simulink model "main_sim_adapt_Gref_SP"  (Simulink 7.2)
settings: Solver=ode2  SolverMode=SingleTasking  StartTime=0.0  StopTime=tsim_max  FixedStep=dtsim  RelTol=1e-3
StopFcn:
  | %mkplt
values from neighbouring files (symbols this model uses):
  aero_surf_qbar_off = get_value('aero_surf_qbar_off')    [setup_claw.m]
  aero_surf_qbar_on = get_value('aero_surf_qbar_on')    [setup_claw.m]
  assertion_time = get_value('assertion_time')    [setup_sim.m]
  att_cmd_select = get_value('att_cmd_select')    [setup_sim.m]
  att_trim_IC = orientation.att'    [setup_claw.m]
  att_type_numbers = cell2mat(struct2cell(att_type))    [setup_constants.m]
  chi_trim_IC = orientation.Vchigam(2)    [setup_claw.m]
  command_time = engage_time + 2.0    [setup_sim.m]
  compute_all_rate_cols = get_value('compute_all_rate_cols')    [setup_claw.m]
  compute_all_vel_cols = get_value('compute_all_vel_cols')    [setup_claw.m]
  da_trim_IC = tmp(1)    [setup_claw.m]
  dc_L2W_IC = orientation.dc_L2W    [setup_claw.m]
  de_trim_IC = tmp(2)    [setup_claw.m]
  dr_trim_IC = tmp(3)    [setup_claw.m]
  dtsim = get_value('dtsim')    [setup_sim.m]
  E_trim_IC = MACH_pos_IC(2)    [setup_claw.m]
  Ed_trim_IC = MACH_vel_IC(2)    [setup_claw.m]
  gain_set = gain_set_next    (= 1)    [setup_claw.m]
  gain_var_struct = rmfield(gain_var_struct,setdiff(fieldnames(gain_var_struct),{'name','size'}))    [setup_claw.m]
  gamma_trim_IC = orientation.Vchigam(3)    [setup_claw.m]
  h_trim_IC = MACH_pos_IC(3)    [setup_claw.m]
  hd_trim_IC = MACH_vel_IC(3)    [setup_claw.m]
  ideal_vel_Kb = MACH_vel_Kb(1)    [setup_sim.m]
  MACH = rmfield(MACH,'vel_throt_lrlim')    [setup_claw.m]
  MACH_att_fb = get_value('MACH_att_fb','onerror',0)    [setup_claw.m]
  MACH_att_int_IC = (1-MACH_att_Kc).*MACH_quat_IC'    [setup_ideal.m]
  MACH_att_Kb = repval(att_kbnom,MACH.att_num_cv)    [setup_claw.m]
  MACH_att_Kc = Ki2Kc(MACH_att_Ki)    [setup_ideal.m]
  MACH_att_Ki = repval(att_fi,MACH.att_num_cv)    [setup_claw.m]
  MACH_gain_mat = vertcat(MACH_gain_mat, this_gain_mat)    [setup_claw.m]
  MACH_mass_IC = obac_params.mass_IC    [setup_claw.m]
  MACH_pos_IC = x_obac_IC(MACH.NEh_idx)    [setup_claw.m]
  MACH_pos_int_IC = (1-MACH_pos_Kc).*MACH_pos_IC' + MACH_vel_IC'./MACH_pos_Kb    [setup_ideal.m]
  MACH_pos_Kb = repval(pos_kbnom,MACH.pos_num_cv)    [setup_claw.m]
  MACH_pos_Kc = Ki2Kc(MACH_pos_Ki)    [setup_ideal.m]
  MACH_pos_Ki = repval(pos_fi,MACH.pos_num_cv)    [setup_claw.m]
  MACH_pqr_Bmat_IC = Bo(MACH.pqr_idx,MACH.pqr_u_idx)    [setup_claw.m]
  MACH_pqr_IC = pqr_trim_IC    [setup_claw.m]
  MACH_pqr_int_IC = (1-MACH_pqr_Kc).*MACH_pqr_IC'    [setup_ideal.m]
  MACH_pqr_Kb = repval(pqr_kbnom,MACH.pqr_num_cv)    [setup_claw.m]
  MACH_pqr_Kc = Ki2Kc(MACH_pqr_Ki)    [setup_ideal.m]
  MACH_pqr_Ki = repval(pqr_fi,MACH.pqr_num_cv)    [setup_claw.m]
  MACH_pqr_u_IC = [ vanes_trim_IC; tvc_trim_IC; rcs_trim_IC ]    [setup_claw.m]
  MACH_quat_IC = quat_trim_IC    [setup_claw.m]
  MACH_throttle_IC = throttle_trim_IC    [setup_claw.m]
  MACH_U_nom_IC = zeros(MACH.num_u,1)    [setup_claw.m]
  MACH_vel_Bmat_IC = MACH_vel_Bmat_IC*inv(vel_perts)    [setup_claw.m]
  MACH_vel_cvdnom_IC = repval(get_value('vel_cvdnom_IC','onerror',MACH_vel_cvdnom_IC),length(MACH_vel_cvdnom_IC))'    [setup_claw.m]
  MACH_vel_IC = orientation.NdEdhd'    [setup_claw.m]
  MACH_vel_int_IC = (1-MACH_vel_Kc).*MACH_vel_IC'    [setup_ideal.m]
  MACH_vel_Kb = repval(vel_kbnom,MACH.vel_num_cv)    [setup_claw.m]
  MACH_vel_Kc = Ki2Kc(MACH_vel_Ki)    [setup_ideal.m]
  MACH_vel_Ki = repval(vel_fi,MACH.vel_num_cv)    [setup_claw.m]
  MACH_vel_uold_IC = [ MACH_quat_IC; MACH_throttle_IC ]    [setup_claw.m]
  N_trim_IC = MACH_pos_IC(1)    [setup_claw.m]
  Nd_trim_IC = MACH_vel_IC(1)    [setup_claw.m]
  obac_params = define_model('obac', get_value('obac_model_type'))    [setup_claw.m]
  pos_cmd_select = get_value('pos_cmd_select')    [setup_sim.m]
  pqr_trim_IC = [ 0 0 0 ]'    [setup_claw.m]
  rate_cmd_select = get_value('rate_cmd_select')    [setup_sim.m]
  rcs_cvddes_thresh = get_value('rcs_cvddes_thresh')    [setup_claw.m]
  reset_camcmd_on_entry = get_value('reset_camcmd_on_entry')    [setup_claw.m]
  throttle_trim_IC = u_obac_IC(MACH.throttle_idx)    [setup_claw.m]
  trac_params = define_model('trac', get_value('trac_model_type','onerror',obac_params.model_type))    [setup_sim.m]
  use_auto_att_type = get_value('use_auto_att_type','onerror',0)    [setup_claw.m]
  use_eow_as_iv = get_value('use_eow_as_iv')    [setup_claw.m]
  use_full_surf_cmd = get_value('use_full_surf_cmd')    [setup_sim.m]
  use_nav = get_value('use_nav')    [setup_claw.m]
  use_NdEdh_pos = get_value('use_NdEdh_pos')    [setup_claw.m]
  use_pos_fltpath_lim = get_value('use_pos_fltpath_lim')    [setup_claw.m]
  use_throt_estimate = get_value('use_throt_estimate')    [setup_claw.m]
  use_variable_mass = get_value('use_variable_mass')    [setup_claw.m]
  use_wind_est = get_value('use_wind_est')    [setup_claw.m]
  V_trim_IC = orientation.Vchigam(1)    [setup_claw.m]
  vel_cmd_ramp_time = get_value('vel_cmd_ramp_time')    [setup_claw.m]
  vel_cmd_select = get_value('vel_cmd_select')    [setup_sim.m]
  x_trac_IC = x_obac_IC    [setup_sim.m]
undefined symbols (not defined in the file or in its folder): accel_cmd, alpha_trim, Am, att_type, B1, bb_ellipsoid, bb_params, Bm, C, constants, cosA, DiscIntNeverNeededParam, DZkx, DZtheta, E_rwy, Ed_cmd, eow_boundary, flag_autoadapt, flag_exsig, flag_uad, full_surf_llim, full_surf_ulim, gam_cmd_descent, gam_cmd_preflare, gamdot_cmd_descent, gamdot_cmd_flare, gamdot_cmd_preflare, Gamtheta, Gamx, hd_cmd, in_error_thresh, in_exsig_vecin, in_exsig_vecout, in_reset_stoptime, in_t_exsig, in_t_timer, in_tadaptoff_forced, in_tadapton_forced, Kb, Kxhat0, Kxnom, Kxstar, max_chi_cmd, max_LOS_rate, max_vel_cmd, min_chi_cmd, min_vel_cmd, modes, N_rwy, Nd_cmd, Nrbf, P, pos, Sig, sinA, target_pos_IC, target_range_blind, target_range_detect, target_range_homing, target_vel_IC ... (+11)
libraries: simulink x44, utility_lib x36, mach_lib x24, model_lib x13, simulink_need_slupdate x8, models x8
(part 1 of 8)
CloseFcn:
  | rtwprivate ssgencode ModelCloseRequest main
settings Model: Creator=E183308  LastModifiedBy=E183308  ModifiedComment=E700252 -- Tue Nov 11 13:33:23 2003 -- Version 1.2477  TunableVars=MACH_U_nom_IC,MACH_gain_mat,MACH_mass_IC,MACH_pos_IC,MACH_pqr_Bmat_IC,MACH_pqr_u_IC,MACH_quat_IC,MACH_throttle_IC,MACH_vel_Bmat_IC,MACH_vel_IC,MACH_vel_cvdnom_IC,MACH_vel_uold_IC  TunableVarsStorageClass=Auto,Auto,Auto,Auto,Auto,Auto,Auto,Auto,Auto,Auto,Auto,Auto  TunableVarsTypeQualifier=,,,,,,,,,,,  BufferReuse=off
settings DataIOCC: LimitDataPoints=off  SaveOutput=off  SaveTime=off  SignalLoggingName=sigsOut
settings OptimizationCC: BlockReduction=off  BooleanDataType=off  BufferReuse=off  EnforceIntegerDowncast=off  FoldNonRolledExpr=off  InitFltsAndDblsToZero=on
settings DebuggingCC: SaveWithParameterizedLinksMsg=none  SignalResolutionControl=TryResolveAllWithWarning  SolverPrmCheckMsg=none  InheritedTsInSrcMsg=none  MultiTaskDSMMsg=warning  MultiTaskCondExecSysMsg=none  StrictBusMsg=ErrorLevel1
settings HardwareCC: TargetEndianess=LittleEndian  TargetHWDeviceType=MATLAB Host  ProdEqTarget=off
settings SFSimCC: SFSimEcho=off
settings RTWCC: SystemTargetFile=rtwsfcn.tlc  TemplateMakefile=rtwsfcn_default_tmf  Description=S-function Target  ProcessScript=rtwsfcn_make_rtw_hook  IncludeERTFirstTime=on
settings STFCustomTargetCC: TargetFcnLib=ansi_tfl_tmw.mat  ModelReferenceCompliant=off  SystemTargetFile=rtwsfcn.tlc
settings CustomProperty: Value=on

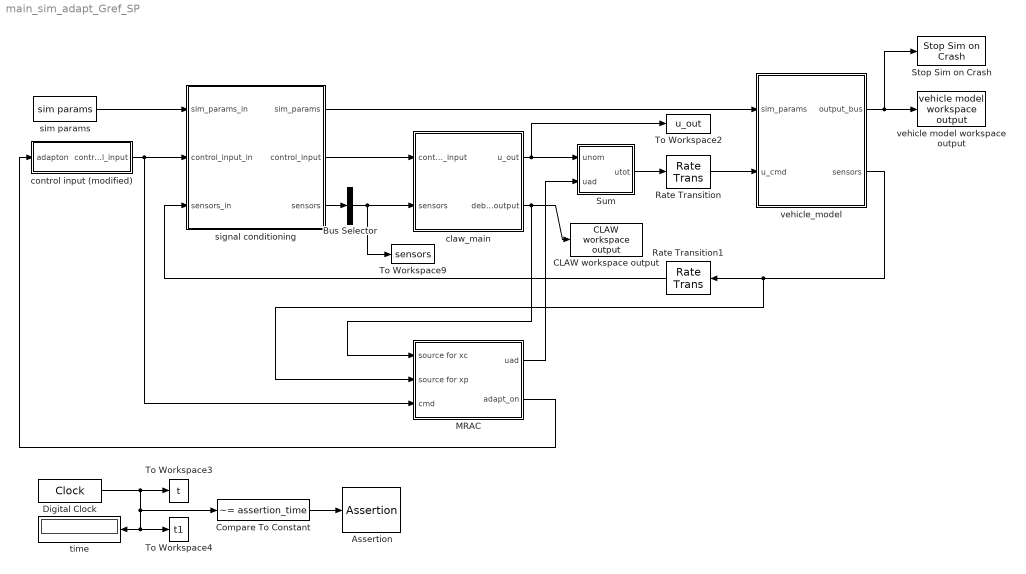
== system main_sim_adapt_Gref_SP ==
  Assertion : Assertion  Enabled=on  AssertionFailFcn=assertioncb  StopWhenAssertionFail=off
  Bus Selector : BusSelector  OutputSignals=pqr,NED_dot,latlonh,e,accels_cg,nav_ok,u_meas,NED_wind,seeker  OutputAsBus=on
  CLAW workspace output : mach_lib/CLAW workspace output  SystemSampleTime=-1
  Compare To Constant : simulink/Logic and Bit Operations/Compare To Constant  SystemSampleTime=-1  relop=~=  const=assertion_time  LogicOutDataTypeMode=boolean  ZeroCross=off
  Digital Clock : DigitalClock  SampleTime=dtsim
  MRAC : Subsystem  SystemSampleTime=dtsim
  Rate Transition : RateTransition  X0=MACH_U_nom_IC
  Rate Transition1 : RateTransition  Orientation=left  OutPortSampleTime=MACH.dt
  Stop Sim on Crash : mach_lib/Stop Sim on Crash  SystemSampleTime=-1
  Sum : Subsystem
  To Workspace2 : ToWorkspace  VariableName=u_out  SampleTime=MACH.dt  SaveFormat=Array
  To Workspace3 : ToWorkspace  VariableName=t  SampleTime=dtsim  SaveFormat=Array
  To Workspace4 : ToWorkspace  VariableName=t1  SampleTime=MACH.dt  SaveFormat=Array
  To Workspace9 : ToWorkspace  VariableName=sensors  SampleTime=MACH.dt  SaveFormat=Array
      settings: MaxDataPoints=Inf
  claw_main : Subsystem  AncestorBlock=mach_lib/claw_main  TreatAsAtomicUnit=on  SystemSampleTime=MACH.dt
  control input (modified) : Subsystem
  signal conditioning : Subsystem
  sim params : mach_lib/sim params  SystemSampleTime=-1
  time : Display
  vehicle model workspace output : mach_lib/vehicle model workspace output  SystemSampleTime=-1
  vehicle_model : Subsystem  TreatAsAtomicUnit=on
  wires:
  Digital Clock/1 -> To Workspace3/1, Compare To Constant/1, time/1, To Workspace4/1
  claw_main/1(u_out) -> Sum/1(unom), To Workspace2/1
  vehicle_model/2(sensors) -> Rate Transition1/1, MRAC/2(source for xp)
  claw_main/2(debug_output) -> CLAW workspace output/1, MRAC/1(source for xc)
  Rate Transition/1 -> vehicle_model/2(u_cmd)
  Bus Selector/1 -> To Workspace9/1, claw_main/2(sensors)
  vehicle_model/1(output_bus) -> vehicle model workspace output/1, Stop Sim on Crash/1
  Rate Transition1/1 -> signal conditioning/3(sensors_in)
  signal conditioning/3(sensors) -> Bus Selector/1
  signal conditioning/2(control_input) -> claw_main/1(control_input)
  sim params/1 -> signal conditioning/1(sim_params_in)
  signal conditioning/1(sim_params) -> vehicle_model/1(sim_params)
  Compare To Constant/1 -> Assertion/1
  MRAC/1(uad) -> Sum/2(uad)
  Sum/1(utot) -> Rate Transition/1
  control input (modified)/1(control_input) -> signal conditioning/2(control_input_in), MRAC/3(cmd)
  MRAC/2(adapt_on) -> control input (modified)/1(adapton)

== system main_sim_adapt_Gref_SP/MRAC ==
  source for xc : Inport
  source for xp : Inport  Port=2
  cmd : Inport  Port=3
  Bus Selector1 : BusSelector  OutputSignals=command  OutputAsBus=on
  Constant : Constant  Value=flag_autoadapt  OutDataType=sfix(16)  OutScaling=2^0
  Enable Adaptation : Subsystem
  Estimate of x : Subsystem
  Force Adaptation : Subsystem
  Model Reference Adaptive Control : Subsystem
  Ref Model : Subsystem
  Reshape : Reshape  OutputDimensionality=Column vector (2-D)
  Selector : Selector  InputPortWidth=4  IndexOptions=Index vector (dialog)  Indices=[2]  OutputSizes=1
  Sum : Sum  Inputs=-|+  OutDataType=sfix(16)  OutScaling=2^0
  Switch : Switch  Threshold=0.5  OutDataType=sfix(16)  OutScaling=2^0
  Terminator : Terminator
  Terminator1 : Terminator
  To Workspace1 : ToWorkspace  VariableName=uad_xm  SampleTime=MACH.dt  SaveFormat=Array
  To Workspace2 : ToWorkspace  VariableName=uad_conv  SampleTime=MACH.dt  SaveFormat=Array
  To Workspace3 : ToWorkspace  VariableName=uad_x  SampleTime=MACH.dt  SaveFormat=Array
  adapt_onoff : Scope
      settings: SaveName=ScopeData26
  command : Scope
      settings: YMin=0  YMax=15  SaveName=ScopeData6
  uad out : Scope
      settings: SaveName=ScopeData15
  uad : Outport  OutDataType=sfix(16)  OutScaling=2^0
  adapt_on : Outport  Port=2  OutDataType=sfix(16)  OutScaling=2^0
  wires:
  Bus Selector1/1 -> Selector/1, Model Reference Adaptive Control/4(r), command/1
  Selector/1 -> Ref Model/2(r)
  cmd/1 -> Bus Selector1/1
  Model Reference Adaptive Control/1(uad) -> uad out/1, uad/1
  Model Reference Adaptive Control/3(Kx_hat) -> Terminator/1
  Model Reference Adaptive Control/4(Theta_hat) -> Terminator1/1
  source for xp/1 -> Estimate of x/2(In2)
  source for xc/1 -> Estimate of x/1(In1)
  Estimate of x/1(x) -> Sum/2, Model Reference Adaptive Control/3(x), Reshape/1, Ref Model/3(x)
  Sum/1 -> Model Reference Adaptive Control/2(e), Enable Adaptation/1(e)
  Model Reference Adaptive Control/2(uad_conv) -> To Workspace2/1
  Ref Model/1(xm) -> Sum/1, To Workspace1/1
  Enable Adaptation/1(adapt on-off) -> Switch/1
  Constant/1 -> Switch/2
  Force Adaptation/1(adapt on-off (forced)) -> Switch/3
  Switch/1 -> Model Reference Adaptive Control/1(adapt on-off), adapt_on/1, adapt_onoff/1, Ref Model/1(enable)
  Reshape/1 -> To Workspace3/1

== system main_sim_adapt_Gref_SP/Sum ==
  unom : Inport
  uad : Inport  Port=2
  Rate Transition1 : RateTransition  OutPortSampleTime=MACH.dt
  Sum : Sum  Inputs=|++  OutDataType=sfix(16)  OutScaling=2^0
  To Workspace1 : ToWorkspace  VariableName=elev_nom  SampleTime=MACH.dt  SaveFormat=Array
  To Workspace2 : ToWorkspace  VariableName=elev_adap  SampleTime=MACH.dt  SaveFormat=Array
  To Workspace9 : ToWorkspace  VariableName=elev_total  SampleTime=MACH.dt  SaveFormat=Array
  get RIE : Selector  InputPortWidth=MACH.num_u  IndexOptions=Index vector (dialog)  Indices=MACH.u_idx.elev  OutputSizes=1
  set RIE : Assignment  IndexOptions=Index vector (dialog)  Indices=MACH.u_idx.elev  OutputSizes=[1 1]
  utot : Outport
  wires:
  unom/1 -> get RIE/1, set RIE/1
  get RIE/1 -> Sum/1, To Workspace1/1
  uad/1 -> Rate Transition1/1
  Sum/1 -> set RIE/2, To Workspace9/1
  set RIE/1 -> utot/1
  Rate Transition1/1 -> To Workspace2/1, Sum/2

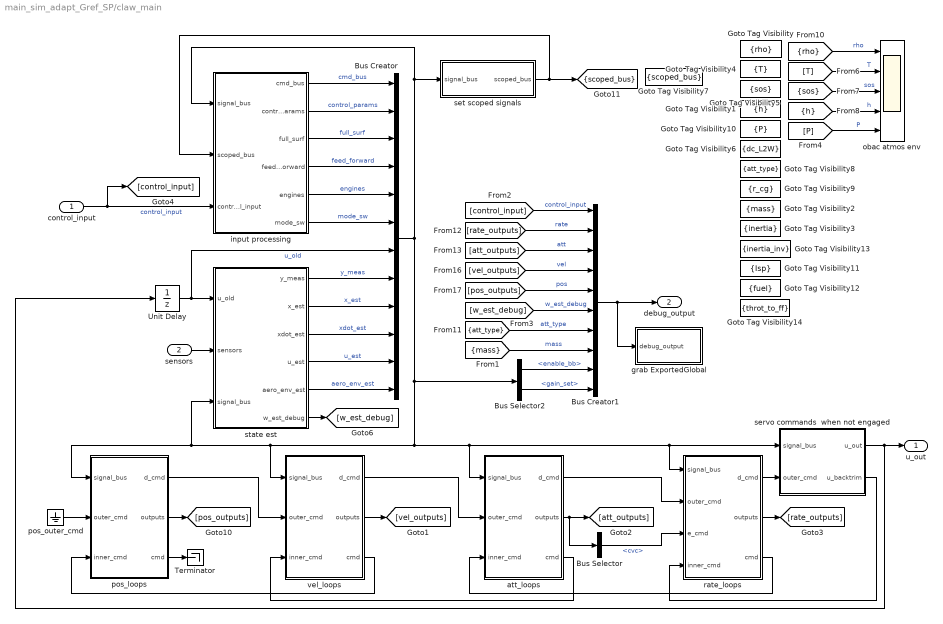
== system main_sim_adapt_Gref_SP/claw_main ==
  control_input : Inport  OutDataType=sfix(16)  OutScaling=2^0
      settings: BusObject=control_input_bus
  sensors : Inport  Port=2  OutDataType=sfix(16)  OutScaling=2^0
  Bus Creator : BusCreator  Inputs=12
  Bus Creator1 : BusCreator  Inputs=10
      settings: BusObject=CLAW_DEBUG_OUTPUT_BUS
  Bus Selector : BusSelector  OutputSignals=cvc
  Bus Selector2 : BusSelector  OutputSignals=control_params.enable_bb,control_params.gain_set
  Goto Tag Visibility : GotoTagVisibility  GotoTag=rho
  Goto Tag Visibility1 : GotoTagVisibility  GotoTag=h
  Goto Tag Visibility10 : GotoTagVisibility  GotoTag=P
  Goto Tag Visibility11 : GotoTagVisibility  GotoTag=Isp
  Goto Tag Visibility12 : GotoTagVisibility  GotoTag=fuel
  Goto Tag Visibility13 : GotoTagVisibility  GotoTag=inertia_inv
  Goto Tag Visibility14 : GotoTagVisibility  GotoTag=throt_to_ff
  Goto Tag Visibility2 : GotoTagVisibility  GotoTag=mass
  Goto Tag Visibility3 : GotoTagVisibility  GotoTag=inertia
  Goto Tag Visibility4 : GotoTagVisibility  GotoTag=T
  Goto Tag Visibility5 : GotoTagVisibility  GotoTag=sos
  Goto Tag Visibility6 : GotoTagVisibility  GotoTag=dc_L2W
  Goto Tag Visibility7 : GotoTagVisibility  GotoTag=scoped_bus
  Goto Tag Visibility8 : GotoTagVisibility  GotoTag=att_type
  Goto Tag Visibility9 : GotoTagVisibility  GotoTag=r_cg
  Terminator : Terminator
  Unit Delay : UnitDelay  X0=MACH_U_nom_IC  SampleTime=-1
  att_loops : Subsystem
  grab ExportedGlobal : Subsystem
  input processing : Subsystem
  obac atmos env : Scope  NumInputPorts=5
      settings: YMin=-5~-5~-5~-5~-5  YMax=5~5~5~5~5  SaveName=ScopeData2
  pos_loops : Subsystem
      settings: RTWSystemCode=Function
  pos_outer_cmd : Ground
  rate_loops : Subsystem
      settings: RTWSystemCode=Function
  servo commands  when not engaged : Subsystem
  set scoped signals : Subsystem
  state est : Subsystem
  vel_loops : Subsystem
      settings: RTWSystemCode=Function
  u_out : Outport  OutDataType=sfix(16)  OutScaling=2^0
  debug_output : Outport  Port=2  OutDataType=sfix(16)  OutScaling=2^0
  tag scope: scoped_bus=scoped
  wires:
  input processing/6(mode_sw) -> Bus Creator/6  "mode_sw"
  input processing/5(engines) -> Bus Creator/5  "engines"
  pos_loops/2(outputs) -> [pos_outputs]
  [pos_outputs] -> Bus Creator1/5  "pos"
  [vel_outputs] -> Bus Creator1/4  "vel"
  [att_outputs] -> Bus Creator1/3  "att"
  [rate_outputs] -> Bus Creator1/2  "rate"
  att_loops/1(d_cmd) -> rate_loops/2(outer_cmd)
  vel_loops/1(d_cmd) -> att_loops/2(outer_cmd)
  rate_loops/1(d_cmd) -> servo commands  when not engaged/2(outer_cmd)
  Bus Creator/1 -> att_loops/1(signal_bus), rate_loops/1(signal_bus), servo commands  when not engaged/1(signal_bus), vel_loops/1(signal_bus), pos_loops/1(signal_bus), state est/3(signal_bus), Bus Selector2/1, input processing/1(signal_bus), set scoped signals/1(signal_bus)
  pos_loops/3(cmd) -> Terminator/1
  att_loops/3(cmd) -> vel_loops/3(inner_cmd)
  rate_loops/3(cmd) -> att_loops/3(inner_cmd)
  pos_loops/1(d_cmd) -> vel_loops/2(outer_cmd)
  vel_loops/2(outputs) -> [vel_outputs]
  att_loops/2(outputs) -> [att_outputs], Bus Selector/1
  rate_loops/2(outputs) -> [rate_outputs]
  Bus Creator1/1 -> debug_output/1, grab ExportedGlobal/1(debug_output)
  Unit Delay/1 -> state est/1(u_old), Bus Creator/7  "u_old"
  sensors/1 -> state est/2(sensors)
  vel_loops/3(cmd) -> pos_loops/3(inner_cmd)
  servo commands  when not engaged/2(u_backtrim) -> rate_loops/4(inner_cmd)
  state est/4(u_est) -> Bus Creator/11  "u_est"
  state est/3(xdot_est) -> Bus Creator/10  "xdot_est"
  state est/2(x_est) -> Bus Creator/9  "x_est"
  state est/1(y_meas) -> Bus Creator/8  "y_meas"
  servo commands  when not engaged/1(u_out) -> u_out/1, Unit Delay/1
  pos_outer_cmd/1 -> pos_loops/2(outer_cmd)
  state est/6(w_est_debug) -> [w_est_debug]
  [w_est_debug] -> Bus Creator1/6  "w_est_debug"
  [att_type] -> Bus Creator1/7  "att_type"
  input processing/2(control_params) -> Bus Creator/2  "control_params"
  [h] -> obac atmos env/4  "h"
  [sos] -> obac atmos env/3  "sos"
  [T] -> obac atmos env/2  "T"
  [rho] -> obac atmos env/1  "rho"
  [P] -> obac atmos env/5  "P"
  state est/5(aero_env_est) -> Bus Creator/12  "aero_env_est"
  input processing/3(full_surf) -> Bus Creator/3  "full_surf"
  input processing/4(feed_forward) -> Bus Creator/4  "feed_forward"
  set scoped signals/1(scoped_bus) -> [scoped_bus], input processing/2(scoped_bus)
  [mass] -> Bus Creator1/8  "mass"
  Bus Selector2/1 -> Bus Creator1/9  "<enable_bb>"
  Bus Selector2/2 -> Bus Creator1/10  "<gain_set>"
  control_input/1 -> input processing/3(control_input), [control_input]  "control_input"
  input processing/1(cmd_bus) -> Bus Creator/1  "cmd_bus"
  [control_input] -> Bus Creator1/1  "control_input"
  Bus Selector/1 -> rate_loops/3(e_cmd)  "<cvc>"

== system main_sim_adapt_Gref_SP/control input (modified) ==
  adapton : Inport
  Add Excitation : Subsystem
  Bus Assignment : BusAssignment  AssignedSignals=command
  control input : Subsystem  AncestorBlock=mach_lib/control input  SystemSampleTime=MACH.dt
  ideal responses : Subsystem  AncestorBlock=model_lib/ideal responses
  control_input : Outport
  wires:
  Bus Assignment/1 -> ideal responses/1(control_input), control_input/1
  Add Excitation/1(Out) -> Bus Assignment/2
  control input/1(control_input) -> Add Excitation/1(In), Bus Assignment/1
  adapton/1 -> Add Excitation/2(Adapt On-Off)

== system main_sim_adapt_Gref_SP/signal conditioning ==
  sim_params_in : Inport  OutDataType=sfix(16)  OutScaling=2^0
  control_input_in : Inport  Port=2  OutDataType=sfix(16)  OutScaling=2^0
  sensors_in : Inport  Port=3  OutDataType=sfix(16)  OutScaling=2^0
  Bus Assignment : BusAssignment  AssignedSignals=full_surf.full_surf_pref
  Bus Selector : BusSelector  OutputSignals=full_surf.full_surf_pref
  Compare To Constant : simulink/Logic and Bit Operations/Compare To Constant  SystemSampleTime=-1  relop=>=  const=0  LogicOutDataTypeMode=boolean  ZeroCross=off
  Compare To Constant1 : simulink/Logic and Bit Operations/Compare To Constant  SystemSampleTime=-1  relop=<=  const=5  LogicOutDataTypeMode=boolean  ZeroCross=off
  Constant : Constant  Value=360  OutDataType=sfix(16)  OutScaling=2^0
  Digital Clock : DigitalClock  SampleTime=MACH.dt
  Gain : Gain  Gain=0  ParameterDataType=sfix(16)  ParameterScaling=2^0  OutDataType=sfix(16)  OutScaling=2^0
  Logical Operator : Logic  AllPortsSameDT=off
  Product : Product  OutDataType=sfix(16)  OutScaling=2^0  RndMeth=Zero
  Sine Wave : Sin  TimeSource=Use external signal  Amplitude=5  Frequency=2*pi  SampleTime=0
  Sum : Sum  Inputs=|++  OutDataType=sfix(16)  OutScaling=2^0
  Sum1 : Sum  Inputs=|+-  OutDataType=sfix(16)  OutScaling=2^0
  get RIE : Selector  InputPortWidth=MACH.num_u  IndexOptions=Index vector (dialog)  Indices=MACH.vane_idx(1)  OutputSizes=1
  set RIE : Assignment  IndexOptions=Index vector (dialog)  Indices=MACH.vane_idx(1)  OutputSizes=[1 1]
  sim_params : Outport  OutDataType=sfix(16)  OutScaling=2^0
  control_input : Outport  Port=2  OutDataType=sfix(16)  OutScaling=2^0
  sensors : Outport  Port=3  OutDataType=sfix(16)  OutScaling=2^0
  wires:
  sim_params_in/1 -> sim_params/1
  control_input_in/1 -> Bus Assignment/1, Bus Selector/1
  sensors_in/1 -> sensors/1
  set RIE/1 -> Bus Assignment/2
  Sum/1 -> set RIE/2
  Bus Selector/1 -> set RIE/1, get RIE/1  "<full_surf_pref>"
  get RIE/1 -> Sum/1
  Digital Clock/1 -> Sum1/1
  Constant/1 -> Sum1/2
  Sum1/1 -> Sine Wave/1, Compare To Constant/1, Compare To Constant1/1
  Compare To Constant/1 -> Logical Operator/1
  Compare To Constant1/1 -> Logical Operator/2
  Logical Operator/1 -> Product/2
  Sine Wave/1 -> Product/1
  Product/1 -> Gain/1
  Bus Assignment/1 -> control_input/1
  Gain/1 -> Sum/2

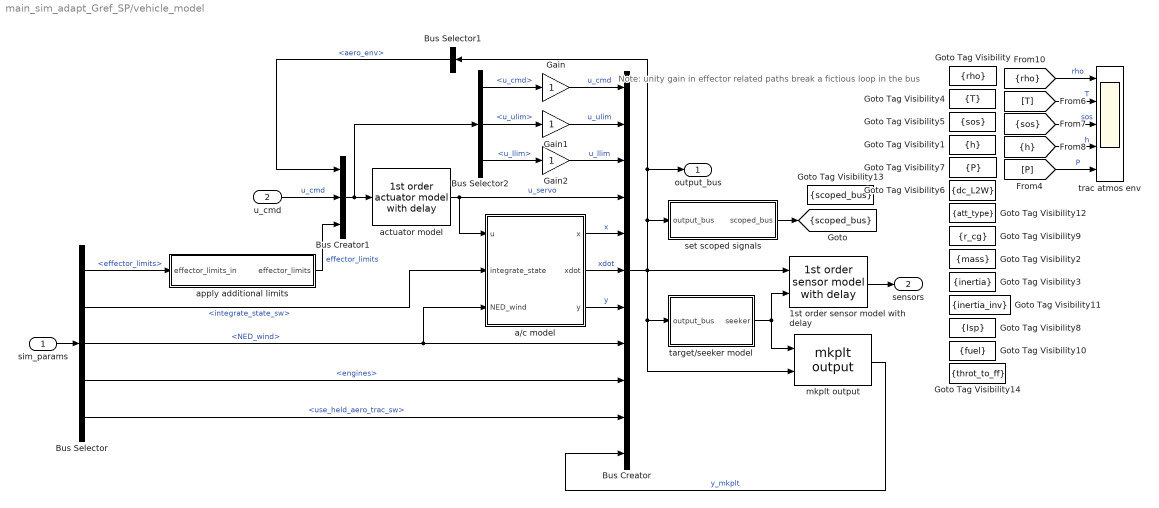
== system main_sim_adapt_Gref_SP/vehicle_model ==
  note: Note: unity gain in effector related paths
      | break a fictious loop in the bus
  sim_params : Inport  OutDataType=sfix(16)  OutScaling=2^0
  u_cmd : Inport  Port=2  OutDataType=sfix(16)  OutScaling=2^0
  1st order sensor model with delay : models/1st order sensor model with delay  SystemSampleTime=-1
  Bus Creator : BusCreator  Inputs=11
  Bus Creator1 : BusCreator  Inputs=3
  Bus Selector : BusSelector  OutputSignals=effector_limits,integrate_state_sw,NED_wind,engines,use_held_aero_trac_sw
  Bus Selector1 : BusSelector  Orientation=left  OutputSignals=y.aero_env
  Bus Selector2 : BusSelector  OutputSignals=u_cmd,effector_limits.u_ulim,effector_limits.u_llim
  Gain : Gain  ParameterDataType=sfix(16)  ParameterScaling=2^0  OutDataType=sfix(16)  OutScaling=2^0
  Gain1 : Gain  ParameterDataType=sfix(16)  ParameterScaling=2^0  OutDataType=sfix(16)  OutScaling=2^0
  Gain2 : Gain  ParameterDataType=sfix(16)  ParameterScaling=2^0  OutDataType=sfix(16)  OutScaling=2^0
  Goto Tag Visibility : GotoTagVisibility  GotoTag=rho
  Goto Tag Visibility1 : GotoTagVisibility  GotoTag=h
  Goto Tag Visibility10 : GotoTagVisibility  GotoTag=fuel
  Goto Tag Visibility11 : GotoTagVisibility  GotoTag=inertia_inv
  Goto Tag Visibility12 : GotoTagVisibility  GotoTag=att_type
  Goto Tag Visibility13 : GotoTagVisibility  GotoTag=scoped_bus
  Goto Tag Visibility14 : GotoTagVisibility  GotoTag=throt_to_ff
  Goto Tag Visibility2 : GotoTagVisibility  GotoTag=mass
  Goto Tag Visibility3 : GotoTagVisibility  GotoTag=inertia
  Goto Tag Visibility4 : GotoTagVisibility  GotoTag=T
  Goto Tag Visibility5 : GotoTagVisibility  GotoTag=sos
  Goto Tag Visibility6 : GotoTagVisibility  GotoTag=dc_L2W
  Goto Tag Visibility7 : GotoTagVisibility  GotoTag=P
  Goto Tag Visibility8 : GotoTagVisibility  GotoTag=Isp
  Goto Tag Visibility9 : GotoTagVisibility  GotoTag=r_cg
  a/c model : Subsystem
  actuator model : models/1st order actuator model with delay  SystemSampleTime=-1
  apply additional limits : Subsystem
  mkplt output : model_lib/mkplt output  SystemSampleTime=-1
  set scoped signals : Subsystem
  target/seeker model : Subsystem
  trac atmos env : Scope  NumInputPorts=5
      settings: YMin=-5~-5~-5~-5~-5  YMax=5~5~5~5~5
  output_bus : Outport  OutDataType=sfix(16)  OutScaling=2^0
  sensors : Outport  Port=2  OutDataType=sfix(16)  OutScaling=2^0
  tag scope: scoped_bus=scoped
  wires:
  actuator model/1 -> a/c model/1(u), Bus Creator/4  "u_servo"
  1st order sensor model with delay/1 -> sensors/1
  Bus Selector/3 -> Bus Creator/8, a/c model/3(NED_wind)  "<NED_wind>"
  [h] -> trac atmos env/4  "h"
  [sos] -> trac atmos env/3  "sos"
  [T] -> trac atmos env/2  "T"
  [rho] -> trac atmos env/1  "rho"
  [P] -> trac atmos env/5  "P"
  target/seeker model/1(seeker) -> mkplt output/1, 1st order sensor model with delay/2
  a/c model/1(x) -> Bus Creator/5  "x"
  a/c model/2(xdot) -> Bus Creator/6  "xdot"
  a/c model/3(y) -> Bus Creator/7  "y"
  Bus Creator/1 -> set scoped signals/1(output_bus), output_bus/1, Bus Selector1/1, target/seeker model/1(output_bus), mkplt output/2, 1st order sensor model with delay/1
  sim_params/1 -> Bus Selector/1
  set scoped signals/1(scoped_bus) -> [scoped_bus]
  Bus Selector/4 -> Bus Creator/9  "<engines>"
  mkplt output/1 -> Bus Creator/11  "y_mkplt"
  Bus Selector/5 -> Bus Creator/10  "<use_held_aero_trac_sw>"
  Bus Creator1/1 -> actuator model/1, Bus Selector2/1
  Bus Selector1/1 -> Bus Creator1/1  "<aero_env>"
  u_cmd/1 -> Bus Creator1/2  "u_cmd"
  Bus Selector2/1 -> Gain/1  "<u_cmd>"
  Bus Selector2/2 -> Gain1/1  "<u_ulim>"
  Bus Selector2/3 -> Gain2/1  "<u_llim>"
  Gain/1 -> Bus Creator/1  "u_cmd"
  Gain1/1 -> Bus Creator/2  "u_ulim"
  Gain2/1 -> Bus Creator/3  "u_llim"
  Bus Selector/2 -> a/c model/2(integrate_state)  "<integrate_state_sw>"
  Bus Selector/1 -> apply additional limits/1(effector_limits_in)  "<effector_limits>"
  apply additional limits/1(effector_limits) -> Bus Creator1/3  "effector_limits"

== system main_sim_adapt_Gref_SP/MRAC/Enable Adaptation ==
  e : Inport
  Abs : Abs  OutDataType=sfix(16)  OutScaling=2^0
  Compare To Zero : simulink/Logic and Bit Operations/Compare To Zero  SystemSampleTime=-1  relop=>  LogicOutDataTypeMode=uint8  ZeroCross=off
  Constant : Constant  Value=in_error_thresh  OutDataType=sfix(16)  OutScaling=2^0
  Data Type Conversion : DataTypeConversion  Orientation=left  OutDataTypeMode=double  OutDataType=sfix(16)  OutScaling=2^0  OutDataTypeStr=double
  Difference : simulink/Discrete/Difference  Orientation=left  SystemSampleTime=-1  ICPrevInput=1  OutMin=[]  OutMax=[]  OutDataType=sfix(16)  OutScaling=2^-10  DoSatur=off
  Is > 0? : simulink/Logic and Bit Operations/Compare To Zero  Orientation=left  SystemSampleTime=-1  relop=>  LogicOutDataTypeMode=boolean  ZeroCross=off
  Memory : Memory  Orientation=left  X0=1  InheritSampleTime=on
  Product : Product  Orientation=left  OutDataType=sfix(16)  OutScaling=2^0  RndMeth=Zero
  Resettable Switch (On with rising signal/ Off with timer) : Subsystem
  Stop Reset Externally : Step  Orientation=left  Time=in_reset_stoptime  Before=1  After=0  SampleTime=0
  Subtract : Sum  Inputs=+-  OutDataType=sfix(16)  OutScaling=2^-10
  Sum of Elements : Sum  Inputs=+  OutDataType=sfix(16)  OutScaling=2^-10
  adapt on? : Scope
      settings: TimeRange=50  YMin=0  YMax=1  SaveName=ScopeData23
  cross threshold : Scope
      settings: TimeRange=50  YMin=0  YMax=1  SaveName=ScopeData22
  cross threshold1 : Scope
      settings: TimeRange=25  YMin=-0.014  YMax=0.002  SaveName=ScopeData31
  reset pulse : Scope
      settings: TimeRange=45  YMin=-1  YMax=1  SaveName=ScopeData20
  reset ready : Scope
      settings: TimeRange=20  YMin=0  YMax=1  SaveName=ScopeData21
  adapt on-off : Outport
  wires:
  Constant/1 -> Subtract/2
  Subtract/1 -> Compare To Zero/1, cross threshold1/1
  e/1 -> Abs/1
  Compare To Zero/1 -> Sum of Elements/1
  Sum of Elements/1 -> Resettable Switch (On with rising signal/ Off with timer)/1(In1), cross threshold/1
  Resettable Switch (On with rising signal/ Off with timer)/1(Out1) -> adapt on-off/1, adapt on?/1
  Resettable Switch (On with rising signal/ Off with timer)/2(reset ready) -> reset ready/1, Memory/1
  Difference/1 -> Is > 0?/1
  Data Type Conversion/1 -> Difference/1
  Memory/1 -> Data Type Conversion/1
  Is > 0?/1 -> Product/1
  Product/1 -> Resettable Switch (On with rising signal/ Off with timer)/2(reset), reset pulse/1
  Stop Reset Externally/1 -> Product/2
  Abs/1 -> Subtract/1

== system main_sim_adapt_Gref_SP/MRAC/Estimate of x ==
  In1 : Inport
  In2 : Inport  Port=2
  Bus Selector : BusSelector  OutputSignals=pqr,e,NED_dot,NED_wind
  Bus Selector22 : BusSelector  OutputSignals=rate.integ
  Constant1 : Constant  Orientation=left  Value=alpha_trim*pi/180  OutDataType=sfix(16)  OutScaling=2^0
  Gain1 : Gain  Gain=-1/(fi*Kb)  ParameterDataType=sfix(16)  ParameterScaling=2^0  OutDataType=sfix(16)  OutScaling=2^0
  Gain3 : Gain  Gain=180/pi  ParameterDataType=sfix(16)  ParameterScaling=2^0  OutDataType=sfix(16)  OutScaling=2^0
  Gain4 : Gain  Gain=180/pi  ParameterDataType=sfix(16)  ParameterScaling=2^0  OutDataType=sfix(16)  OutScaling=2^0
  Gain6 : Gain  Gain=180/pi  ParameterDataType=sfix(16)  ParameterScaling=2^0  OutDataType=sfix(16)  OutScaling=2^0
  Mux : Mux  Inputs=2
  Mux1 : Mux  Inputs=2
  Product : Product  Multiplication=Matrix(*)  OutDataType=sfix(16)  OutScaling=2^0  SaturateOnIntegerOverflow=on  OutDataTypeStr=Inherit: Same as first input
  Reshape : Reshape  OutputDimensionality=Customize  OutputDimensions=[3,3]
  Reshape1 : Reshape  OutputDimensionality=Column vector (2-D)
  Selector1 : Selector  InputPortWidth=3  IndexOptions=Index vector (dialog)  Indices=[2]  OutputSizes=1
  Selector2 : Selector  InputPortWidth=3  IndexOptions=Index vector (dialog)  Indices=[2]  OutputSizes=1
  Sensor : StateSpace  A=-diag([100 100])  B=diag([100 100])  C=eye(2)  D=zeros(2,2)
  Sum1 : Sum  Inputs=|++  OutDataType=sfix(16)  OutScaling=2^0  SaturateOnIntegerOverflow=on
  Sum2 : Sum  Orientation=left  Inputs=|-+  OutDataType=sfix(16)  OutScaling=2^0
  Terminator2 : Terminator
  Terminator3 : Terminator
  Transport Delay : TransportDelay  DelayTime=0.02
  alpha : Scope
      settings: YMin=-1  YMax=1  SaveName=ScopeData16
  del alpha : Scope
      settings: YMin=-1  YMax=1  SaveName=ScopeData25
  e2dc : utility_lib/e2dc  SystemSampleTime=-1
  q : Scope
      settings: SaveName=ScopeData11
  uvw_rw2Vab : utility_lib/uvw_rw2Vab  SystemSampleTime=-1
  xc : Scope
      settings: SaveName=ScopeData10
  x : Outport
  wires:
  Bus Selector/1 -> Selector1/1  "<pqr>"
  Bus Selector/2 -> e2dc/1  "<e>"
  Bus Selector22/1 -> Selector2/1  "<integ>"
  Selector2/1 -> Gain1/1  "xc"
  e2dc/1 -> Reshape/1
  uvw_rw2Vab/2 -> Gain6/1, Sum2/2  "alpha"
  Gain6/1 -> alpha/1
  Sum1/1 -> Product/2
  Bus Selector/3 -> Sum1/1  "<NED_dot>"
  Bus Selector/4 -> Sum1/2  "<NED_wind>"
  Product/1 -> uvw_rw2Vab/1
  Reshape/1 -> Product/1
  uvw_rw2Vab/1 -> Terminator2/1
  uvw_rw2Vab/3 -> Terminator3/1
  Gain3/1 -> q/1
  Selector1/1 -> Gain3/1, Mux/1  "q"
  Sum2/1 -> Gain4/1, Mux/2
  Constant1/1 -> Sum2/1
  Gain4/1 -> del alpha/1
  In1/1 -> Bus Selector22/1
  Mux/1 -> Sensor/1
  In2/1 -> Bus Selector/1
  Gain1/1 -> xc/1, Mux1/1
  Mux1/1 -> Reshape1/1
  Reshape1/1 -> x/1
  Sensor/1 -> Transport Delay/1
  Transport Delay/1 -> Mux1/2

== system main_sim_adapt_Gref_SP/MRAC/Force Adaptation ==
  Sum1 : Sum  Inputs=|+-  OutDataType=sfix(16)  OutScaling=2^0
  adapt off (forced) : Step  Time=in_tadaptoff_forced  SampleTime=0
  adapt on (forced) : Step  Time=in_tadapton_forced  SampleTime=0
  adapt on-off (forced) : Outport
  wires:
  adapt on (forced)/1 -> Sum1/1
  adapt off (forced)/1 -> Sum1/2
  Sum1/1 -> adapt on-off (forced)/1

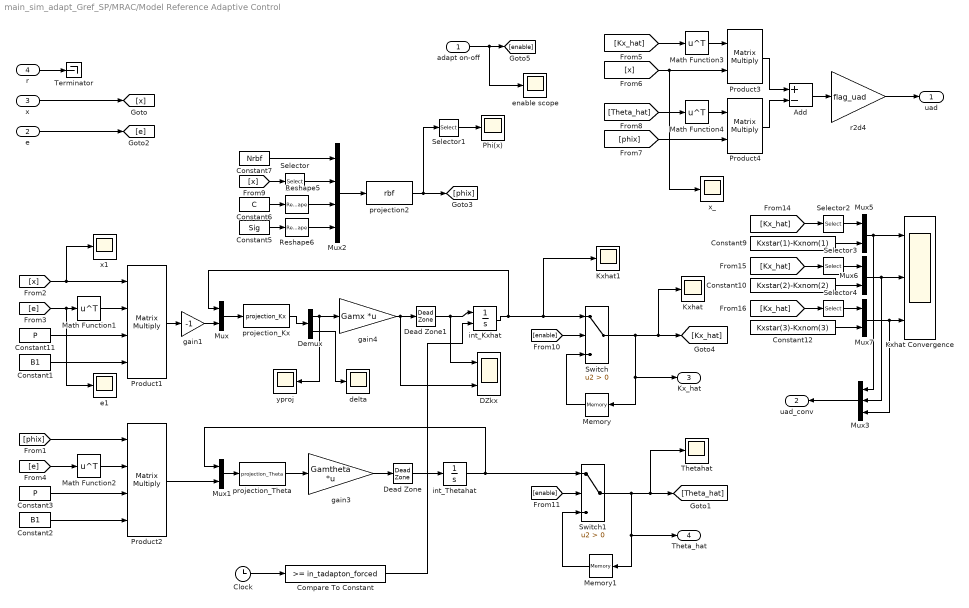
== system main_sim_adapt_Gref_SP/MRAC/Model Reference Adaptive Control ==
  adapt on-off : Inport  OutDataType=sfix(16)  OutScaling=2^0
  e : Inport  Port=2  OutDataType=sfix(16)  OutScaling=2^0
  x : Inport  Port=3  OutDataType=sfix(16)  OutScaling=2^0
  r : Inport  Port=4  OutDataType=sfix(16)  OutScaling=2^0
  Add : Sum  Inputs=+-  OutDataType=sfix(16)  OutScaling=2^-10
  Clock : Clock
      settings: Decimation=10
  Compare To Constant : simulink/Logic and Bit Operations/Compare To Constant  SystemSampleTime=-1  relop=>=  const=in_tadapton_forced  LogicOutDataTypeMode=boolean  ZeroCross=off
  Constant1 : Constant  Value=B1  OutDataType=sfix(16)  OutScaling=2^0
  Constant10 : Constant  Value=Kxstar(2)-Kxnom(2)  OutDataType=sfix(16)  OutScaling=2^0
  Constant11 : Constant  Value=P  OutDataType=sfix(16)  OutScaling=2^0
  Constant12 : Constant  Value=Kxstar(3)-Kxnom(3)  OutDataType=sfix(16)  OutScaling=2^0
  Constant2 : Constant  Value=B1  OutDataType=sfix(16)  OutScaling=2^0
  Constant3 : Constant  Value=P  OutDataType=sfix(16)  OutScaling=2^0
  Constant5 : Constant  Value=Sig  OutDataType=sfix(16)  OutScaling=2^0
  Constant6 : Constant  Value=C  OutDataType=sfix(16)  OutScaling=2^0
  Constant7 : Constant  Value=Nrbf  OutDataType=sfix(16)  OutScaling=2^0
  Constant9 : Constant  Value=Kxstar(1)-Kxnom(1)  OutDataType=sfix(16)  OutScaling=2^0
  DZkx : Scope  NumInputPorts=2
      settings: TimeRange=15  YMin=-10000~-10000  YMax=70000~70000  SaveName=ScopeData14
  Dead Zone : DeadZone  LowerValue=-DZtheta  UpperValue=DZtheta  SaturateOnIntegerOverflow=on
  Dead Zone1 : DeadZone  LowerValue=-DZkx  UpperValue=DZkx  SaturateOnIntegerOverflow=on
  Demux : Demux  Outputs=[3 3]
  Kxhat : Scope
      settings: TimeRange=6  YMin=-75  YMax=225  SaveName=ScopeData4
  Kxhat Convergence : Scope  NumInputPorts=3
      settings: TimeRange=45  YMin=-50~-20~-50  YMax=150~140~200  SaveName=ScopeData13
  Kxhat1 : Scope
      settings: TimeRange=6  YMin=-15  YMax=45  SaveName=ScopeData28
  Math Function{1..4} (4 alike) : Math  Operator=transpose  OutDataType=sfix(16)  OutScaling=2^0  SaturateOnIntegerOverflow=on
  Memory : Memory  Orientation=left  X0=Kxhat0  InheritSampleTime=on
  Memory1 : Memory  Orientation=left  X0=Thetahat0  InheritSampleTime=on
  Mux : Mux  Inputs=2
  Mux1 : Mux  Inputs=2
  Mux2 : Mux
  Mux3 : Mux  Orientation=left  Inputs=3
  Mux5 : Mux  Inputs=[1 1]
  Mux6 : Mux  Inputs=[1 1]
  Mux7 : Mux  Inputs=[1 1]
  Phi(x) : Scope
      settings: TimeRange=40  YMin=-0.05  YMax=0.9  SaveName=ScopeData12
  Product1 : Product  Inputs=4  Multiplication=Matrix(*)  OutDataType=sfix(16)  OutScaling=2^0  RndMeth=Zero
  Product2 : Product  Inputs=4  Multiplication=Matrix(*)  OutDataType=sfix(16)  OutScaling=2^0  RndMeth=Zero
  Product3 : Product  Multiplication=Matrix(*)  OutDataType=sfix(16)  OutScaling=2^0  RndMeth=Zero
  Product4 : Product  Multiplication=Matrix(*)  OutDataType=sfix(16)  OutScaling=2^0  RndMeth=Zero
  Reshape5 : Reshape  OutputDimensions=[1,Nrbf]
  Reshape6 : Reshape  OutputDimensions=[Nrbf,1]
  Selector : Selector  InputPortWidth=nx  IndexOptions=Index vector (dialog)  Indices=3  OutputSizes=1
  Selector1 : Selector  InputPortWidth=11  IndexOptions=Select all  Indices=5  OutputSizes=1
  Selector2 : Selector  InputPortWidth=3  IndexOptions=Index vector (dialog)  Indices=1  OutputSizes=1
  Selector3 : Selector  InputPortWidth=3  IndexOptions=Index vector (dialog)  Indices=2  OutputSizes=1
  Selector4 : Selector  InputPortWidth=3  IndexOptions=Index vector (dialog)  Indices=3  OutputSizes=1
  Switch : Switch  Criteria=u2 > Threshold
  Switch1 : Switch  Criteria=u2 > Threshold
  Terminator : Terminator
  Thetahat : Scope
      settings: TimeRange=40  YMin=-0.3  YMax=0.4  SaveName=ScopeData7
  delta : Scope
      settings: TimeRange=40  YMin=-0.05  YMax=0.9
  e1 : Scope
      settings: TimeRange=30  YMin=-400  YMax=500  SaveName=ScopeData19
  enable scope : Scope
      settings: TimeRange=40  YMin=-0.05  YMax=0.9  SaveName=ScopeData17
  gain1 : Gain  Gain=-1  ParameterDataType=sfix(16)  ParameterScaling=2^0  OutDataType=sfix(16)  OutScaling=2^0
  gain3 : Gain  Gain=Gamtheta  Multiplication=Matrix(K*u)  ParameterDataType=sfix(16)  ParameterScaling=2^0  OutDataType=sfix(16)  OutScaling=2^0
  gain4 : Gain  Gain=Gamx  Multiplication=Matrix(K*u)  ParameterDataType=sfix(16)  ParameterScaling=2^0  OutDataType=sfix(16)  OutScaling=2^0
  int_Kxhat : Integrator  ExternalReset=rising  InitialCondition=Kxhat0
  int_Thetahat : Integrator  InitialCondition=Thetahat0
  projection2 : MATLABFcn  MATLABFcn=rbf  OutputDimensions=[Nrbf,1]  Output1D=off
  projection_Kx : MATLABFcn  MATLABFcn=projection_Kx
  projection_Theta : MATLABFcn  MATLABFcn=projection_Theta
  r2d4 : Gain  Gain=flag_uad  ParameterDataType=sfix(16)  ParameterScaling=2^0  OutDataType=sfix(16)  OutScaling=2^0
  x1 : Scope
      settings: TimeRange=25  YMin=-0.04  YMax=0.035  SaveName=ScopeData18
  x_ : Scope
      settings: TimeRange=40  YMin=-0.05  YMax=0.15  SaveName=ScopeData21
  yproj : Scope
      settings: TimeRange=40  YMin=-0.05  YMax=0.9  SaveName=ScopeData2
  uad : Outport  OutDataType=sfix(16)  OutScaling=2^0  InitialOutput=0
  uad_conv : Outport  Orientation=left  Port=2  OutDataType=sfix(16)  OutScaling=2^0  InitialOutput=0
  Kx_hat : Outport  Port=3  OutDataType=sfix(16)  OutScaling=2^0  InitialOutput=0
  Theta_hat : Outport  Port=4  OutDataType=sfix(16)  OutScaling=2^0  InitialOutput=0
  wires:
  Memory/1 -> Switch/3
  Memory1/1 -> Switch1/3
  adapt on-off/1 -> enable scope/1, [enable]
  [enable] -> Switch/2
  Switch/1 -> Memory/1, Kx_hat/1, Kxhat/1, [Kx_hat]
  [enable] -> Switch1/2
  Switch1/1 -> Memory1/1, Theta_hat/1, Thetahat/1, [Theta_hat]
  Demux/2 -> delta/1
  Demux/1 -> yproj/1, gain4/1
  projection_Kx/1 -> Demux/1
  gain4/1 -> DZkx/2, Dead Zone1/1
  Dead Zone1/1 -> DZkx/1, int_Kxhat/1
  Mux7/1 -> Kxhat Convergence/3, Mux3/3
  Mux6/1 -> Kxhat Convergence/2, Mux3/2
  Mux5/1 -> Kxhat Convergence/1, Mux3/1
  Constant12/1 -> Mux7/2
  Selector4/1 -> Mux7/1
  [Kx_hat] -> Selector4/1
  Constant10/1 -> Mux6/2
  Selector3/1 -> Mux6/1
  [Kx_hat] -> Selector3/1
  Constant9/1 -> Mux5/2
  Selector2/1 -> Mux5/1
  [Kx_hat] -> Selector2/1
  Dead Zone/1 -> int_Thetahat/1
  Selector1/1 -> Phi(x)/1
  r2d4/1 -> uad/1
  Selector/1 -> Mux2/2
  Reshape6/1 -> Mux2/4
  Reshape5/1 -> Mux2/3
  [x] -> Selector/1
  Constant7/1 -> Mux2/1
  projection2/1 -> Selector1/1, [phix]
  Mux2/1 -> projection2/1
  Constant5/1 -> Reshape6/1
  Constant6/1 -> Reshape5/1
  Add/1 -> r2d4/1
  Product4/1 -> Add/2
  Product3/1 -> Add/1
  [phix] -> Product4/2
  Math Function4/1 -> Product4/1
  [Theta_hat] -> Math Function4/1
  Mux1/1 -> projection_Theta/1
  gain3/1 -> Dead Zone/1
  projection_Theta/1 -> gain3/1
  Constant2/1 -> Product2/4
  Constant3/1 -> Product2/3
  Math Function2/1 -> Product2/2
  [phix] -> Product2/1
  Product2/1 -> Mux1/2
  [e] -> Math Function2/1
  Mux/1 -> projection_Kx/1
  gain1/1 -> Mux/2
  x/1 -> [x]
  Constant1/1 -> Product1/4
  Constant11/1 -> Product1/3
  Math Function1/1 -> Product1/2
  [x] -> x1/1, Product1/1
  Product1/1 -> gain1/1
  [x] -> Product3/2, x_/1
  Math Function3/1 -> Product3/1
  [Kx_hat] -> Math Function3/1
  [e] -> e1/1, Math Function1/1
  e/1 -> [e]
  r/1 -> Terminator/1
  int_Kxhat/1 -> Mux/1, Switch/1, Kxhat1/1
  int_Thetahat/1 -> Switch1/1, Mux1/1
  Mux3/1 -> uad_conv/1
  Clock/1 -> Compare To Constant/1
  Compare To Constant/1 -> int_Kxhat/2

== system main_sim_adapt_Gref_SP/MRAC/Ref Model ==
  enable : Inport  OutDataType=sfix(16)  OutScaling=2^0
  r : Inport  Port=2  OutDataType=sfix(16)  OutScaling=2^0
  x : Inport  Port=3  OutDataType=sfix(16)  OutScaling=2^0
  Am : Gain  Orientation=left  Gain=Am  Multiplication=Matrix(K*u)  ParameterDataType=sfix(16)  ParameterScaling=2^0  OutDataType=sfix(16)  OutScaling=2^0
  Bm : Gain  Gain=Bm  Multiplication=Matrix(K*u)  ParameterDataType=sfix(16)  ParameterScaling=2^0  OutDataType=sfix(16)  OutScaling=2^0
  Clock : Clock
      settings: Decimation=10
  Compare To Constant : simulink/Logic and Bit Operations/Compare To Constant  SystemSampleTime=-1  relop=>=  const=in_tadapton_forced  LogicOutDataTypeMode=boolean  ZeroCross=off
  Constant : Constant  Value=[0 0 0]  OutDataType=sfix(16)  OutScaling=2^0
  Constant1 : Constant  Value="[0.0215    0.0052    0.0041]"  OutDataType=sfix(16)  OutScaling=2^0
  Integrator : Integrator  ExternalReset=rising  InitialConditionSource=external  InitialCondition=xm0
  Memory : Memory  InheritSampleTime=on
  Sum2 : Sum  Inputs=|++  OutDataType=sfix(16)  OutScaling=2^0
  Switch : Switch  Threshold=in_tadapton_forced  OutDataType=sfix(16)  OutScaling=2^0
  Terminator : Terminator
  Terminator1 : Terminator
  xm : Outport  OutDataType=sfix(16)  OutScaling=2^0
  wires:
  r/1 -> Bm/1
  Integrator/1 -> Am/1, xm/1
  Am/1 -> Sum2/2
  Sum2/1 -> Integrator/1
  Bm/1 -> Sum2/1
  Constant1/1 -> Switch/1
  Constant/1 -> Switch/3
  Clock/1 -> Switch/2, Compare To Constant/1
  Switch/1 -> Terminator/1
  Compare To Constant/1 -> Terminator1/1
  enable/1 -> Memory/1
  x/1 -> Integrator/3
  Memory/1 -> Integrator/2

== system main_sim_adapt_Gref_SP/claw_main/att_loops ==
  signal_bus : Inport  OutDataType=sfix(16)  OutScaling=2^0
  outer_cmd : Inport  Port=2  OutDataType=sfix(16)  OutScaling=2^0
  inner_cmd : Inport  Port=3  OutDataType=sfix(16)  OutScaling=2^0
  Bus Creator : BusCreator  Inputs=7
  Bus Selector : BusSelector  OutputSignals=control_params.limit_pqr_cmd,x_est.uvw,x_est.e
  Bus Selector4 : BusSelector  OutputSignals=feed_forward.att_ff,mode_sw.int_reset_sw,control_params.att_desdyn
  Demux1 : Demux  Outputs=[ MACH.att_num_u MACH.num_u_throt ]
  Mux2 : Mux  Inputs=2
  P+I+AW+TRIM Control : Subsystem
  compute trim : Subsystem
  dc2mba : utility_lib/dc2mba  SystemSampleTime=-1
  dc2tiltcam : utility_lib/dc2tiltcam  SystemSampleTime=-1
  dc2ypr : utility_lib/dc2ypr  SystemSampleTime=-1
  dyn inv : Subsystem
  e2dc : utility_lib/e2dc  SystemSampleTime=-1
  low pass filter : Subsystem
  select att cmd : Subsystem
  d_cmd : Outport  OutDataType=sfix(16)  OutScaling=2^0
  outputs : Outport  Port=2  OutDataType=sfix(16)  OutScaling=2^0
  cmd : Outport  Port=3  OutDataType=sfix(16)  OutScaling=2^0
  wires:
  Mux2/1 -> d_cmd/1
  [throt] -> Mux2/2
  P+I+AW+TRIM Control/2(int state) -> Bus Creator/2  "integ"
  dyn inv/3(cvdex) -> [cvdex], Bus Creator/1  "cvdex"
  Bus Selector/3 -> select att cmd/1(e_current), dyn inv/3(e nom), [cv], P+I+AW+TRIM Control/1(cv)  "<e>"
  outer_cmd/1 -> select att cmd/3(outer cmd)
  P+I+AW+TRIM Control/1(cvdot des) -> dyn inv/4(e dot des)
  [cvdex] -> P+I+AW+TRIM Control/4(cvdot extra)
  dyn inv/1(Bmat) -> compute trim/2(Bmat)
  [trim] -> P+I+AW+TRIM Control/5(trim)
  signal_bus/1 -> Bus Selector/1, select att cmd/4(signal_bus), Bus Selector4/1, low pass filter/2(signal_bus)
  compute trim/1(trim) -> [trim]
  select att cmd/2(throt_cmd) -> [throt]
  [cvc] -> Bus Creator/3, e2dc/1  "cvc"
  Bus Creator/1 -> outputs/1
  inner_cmd/1 -> Demux1/1
  Demux1/1 -> compute trim/1(inner cmd)
  Demux1/2 -> [throt_inner]
  dc2tiltcam/1 -> Bus Creator/5  "tiltcam_cmds"
  [cv] -> Bus Creator/4  "cv"
  e2dc/1 -> dc2tiltcam/1, dc2ypr/1, dc2mba/1
  dc2ypr/1 -> Bus Creator/6  "rpy_cmds"
  dc2mba/1 -> Bus Creator/7  "mab_cmds"
  Bus Selector/2 -> dyn inv/2(uvw)  "<uvw>"
  Bus Selector4/3 -> P+I+AW+TRIM Control/7(x0)  "<att_desdyn>"
  select att cmd/3(cmd) -> cmd/1
  dyn inv/2(pqr) -> Mux2/1, compute trim/3(cmd)
  Bus Selector4/2 -> P+I+AW+TRIM Control/6(reset)  "<int_reset_sw>"
  Bus Selector/1 -> dyn inv/1(limit_pqr_cmd)  "<limit_pqr_cmd>"
  [throt_inner] -> select att cmd/2(throt_current)
  select att cmd/1(e_cmd) -> low pass filter/1(e_cmd), [cvc]
  low pass filter/1(cv cmd) -> P+I+AW+TRIM Control/2(cv cmd)
  low pass filter/2(cvd ff) -> P+I+AW+TRIM Control/3(cvd ff)
  Bus Selector4/1 -> low pass filter/3(att_ff)  "<att_ff>"

== system main_sim_adapt_Gref_SP/claw_main/grab ExportedGlobal ==
  debug_output : Inport  OutDataType=sfix(16)  OutScaling=2^0
  Terminator{1..4,6} (5 alike) : Terminator
  grab cv variables : Subsystem
  grab cvcmd variables : Subsystem
  grab cvdex variables : Subsystem
  grab integrator variables : Subsystem
  grab w_est variables : Subsystem
  wires:
  debug_output/1 -> grab cv variables/1(In1), grab w_est variables/1(In1), grab cvcmd variables/1(In1), grab integrator variables/1(In1), grab cvdex variables/1(In1)
  grab cvdex variables/1(Out1) -> Terminator1/1
  grab integrator variables/1(Out1) -> Terminator2/1
  grab cvcmd variables/1(Out1) -> Terminator3/1
  grab cv variables/1(Out1) -> Terminator4/1
  grab w_est variables/1(Out1) -> Terminator6/1

== system main_sim_adapt_Gref_SP/claw_main/input processing ==
  signal_bus : Inport  OutDataType=sfix(16)  OutScaling=2^0
  scoped_bus : Inport  Port=2  OutDataType=sfix(16)  OutScaling=2^0
  control_input : Inport  Port=3  OutDataType=sfix(16)  OutScaling=2^0
  Bus Selector2 : BusSelector  OutputSignals=full_surf
  Bus Selector3 : BusSelector  OutputSignals=engines,mode_sw,command
  Bus Selector4 : BusSelector  OutputSignals=u_old,y_meas.u_meas
  mode dependent stick processing : Subsystem
  modify limits and apply to direct commands : Subsystem
  select att_type : Subsystem
  set control parameters : Subsystem
  cmd_bus : Outport  OutDataType=sfix(16)  OutScaling=2^0
  control_params : Outport  Port=2  OutDataType=sfix(16)  OutScaling=2^0
  full_surf : Outport  Port=3  OutDataType=sfix(16)  OutScaling=2^0
  feed_forward : Outport  Port=4  OutDataType=sfix(16)  OutScaling=2^0
  engines : Outport  Port=5  OutDataType=sfix(16)  OutScaling=2^0
  mode_sw : Outport  Port=6  OutDataType=sfix(16)  OutScaling=2^0
  wires:
  Bus Selector3/1 -> engines/1  "<engines>"
  mode dependent stick processing/1(cmd_bus) -> cmd_bus/1
  Bus Selector3/3 -> mode dependent stick processing/1(command)  "<command>"
  set control parameters/1(control_params) -> control_params/1
  Bus Selector4/1 -> modify limits and apply to direct commands/1(u_old)  "<u_old>"
  Bus Selector2/1 -> modify limits and apply to direct commands/3(full_surf_in)  "<full_surf>"
  modify limits and apply to direct commands/1(full_surf) -> full_surf/1, set control parameters/2(full_surf)
  control_input/1 -> Bus Selector3/1, Bus Selector2/1
  signal_bus/1 -> set control parameters/1(signal_bus), Bus Selector4/1, mode dependent stick processing/2(signal_bus), select att_type/3(signal_bus)
  mode dependent stick processing/2(feed_forward) -> feed_forward/1
  Bus Selector3/2 -> select att_type/2(mode_sw_in)  "<mode_sw>"
  scoped_bus/1 -> select att_type/1(scoped_bus)
  select att_type/1(mode_sw) -> mode_sw/1
  Bus Selector4/2 -> modify limits and apply to direct commands/2(u_meas)  "<u_meas>"

== system main_sim_adapt_Gref_SP/claw_main/pos_loops ==
  signal_bus : Inport  OutDataType=sfix(16)  OutScaling=2^0
  outer_cmd : Inport  Port=2  OutDataType=sfix(16)  OutScaling=2^0
  inner_cmd : Inport  Port=3  OutDataType=sfix(16)  OutScaling=2^0
  Bus Creator : BusCreator  Inputs=5
  Bus Selector : BusSelector  OutputSignals=feed_forward.pos_ff,mode_sw.int_reset_sw,control_params.pos_desdyn,y_meas.dc_fltpath
  Bus Selector1 : BusSelector  OutputSignals=x_est.NEh
  Mux : Mux  Inputs=[3 1 ]
  P+I+AW+TRIM Control : mach_lib/P+I+AW+TRIM Control  SystemSampleTime=-1
  Product : Product  Multiplication=Matrix(*)  OutDataType=sfix(16)  OutScaling=2^0  RndMeth=Zero
  Selector1 : Selector  InputPortWidth=4  IndexOptions=Index vector (dialog)  Indices=[1 2 4]  OutputSizes=1
  Selector3 : Selector  InputPortWidth=4  IndexOptions=Index vector (dialog)  Indices=[1 2 4 3]  OutputSizes=1
  compute trim : Subsystem
  limiter : Subsystem
  select pos cmd : Subsystem
  d_cmd : Outport  OutDataType=sfix(16)  OutScaling=2^0
  outputs : Outport  Port=2  OutDataType=sfix(16)  OutScaling=2^0
  cmd : Outport  Port=3  OutDataType=sfix(16)  OutScaling=2^0
  wires:
  [camcmd] -> Mux/2
  Mux/1 -> Selector3/1
  select pos cmd/1(NEh_cmd) -> P+I+AW+TRIM Control/2, [cvc]
  Bus Selector1/1 -> P+I+AW+TRIM Control/1, [cv], select pos cmd/1(NEh_current)  "<NEh>"
  signal_bus/1 -> Bus Selector/1, select pos cmd/3(signal_bus), Bus Selector1/1, limiter/2(signal_bus)
  compute trim/1(trim) -> [trim]
  inner_cmd/1 -> Selector1/1
  Selector1/1 -> compute trim/1(inner cmd), limiter/1(vel_inner_cmd)
  outer_cmd/1 -> select pos cmd/2(outer cmd)
  select pos cmd/3(cmd) -> cmd/1
  Selector3/1 -> d_cmd/1
  [cvc] -> Bus Creator/3  "cvc"
  [cv] -> Bus Creator/4  "cv"
  [trim] -> P+I+AW+TRIM Control/5
  [cvdex] -> P+I+AW+TRIM Control/4
  Bus Selector/2 -> P+I+AW+TRIM Control/6  "<int_reset_sw>"
  Bus Selector/3 -> P+I+AW+TRIM Control/7  "<pos_desdyn>"
  limiter/1(cvd_des) -> Mux/1, compute trim/2(cmd)
  P+I+AW+TRIM Control/1 -> limiter/3(cvd_des_in)
  [cvdex] -> Product/2
  P+I+AW+TRIM Control/2 -> Bus Creator/2  "integ"
  Bus Creator/1 -> outputs/1
  Bus Selector/4 -> Product/1  "<dc_fltpath>"
  Product/1 -> Bus Creator/5  "cvdex_fltpath"
  limiter/2(cvd_extra) -> Bus Creator/1, [cvdex]  "cvdex"
  Bus Selector/1 -> P+I+AW+TRIM Control/3  "<pos_ff>"
  select pos cmd/2(cam_cmd) -> [camcmd]
